simulink model "PMSM_RobotKinematics"  (R2018b)
settings: Solver=VariableStepAuto  StartTime=0.0  StopTime=0.2  FixedStep=Ts  RelTol=1e-4  EnableMultiTasking=on
PreLoadFcn:
  | run('Arm6Assembly_DataFile.m');
model workspace: external: MAT-File E:\SixRobotArm\Simscape_Simulation\StepFile\Arm6Assembly_DataFile.mat (data not in the file)
values from neighbouring files (symbols this model uses):
  smiData =     [Arm6SimscapeData.mat]
undefined symbols (not defined in the file or in its folder): X, Y, Z
libraries: sm_lib x36, fl_lib x25, nesl_utility x19, simulink_extras x7
(part 2 of 4)

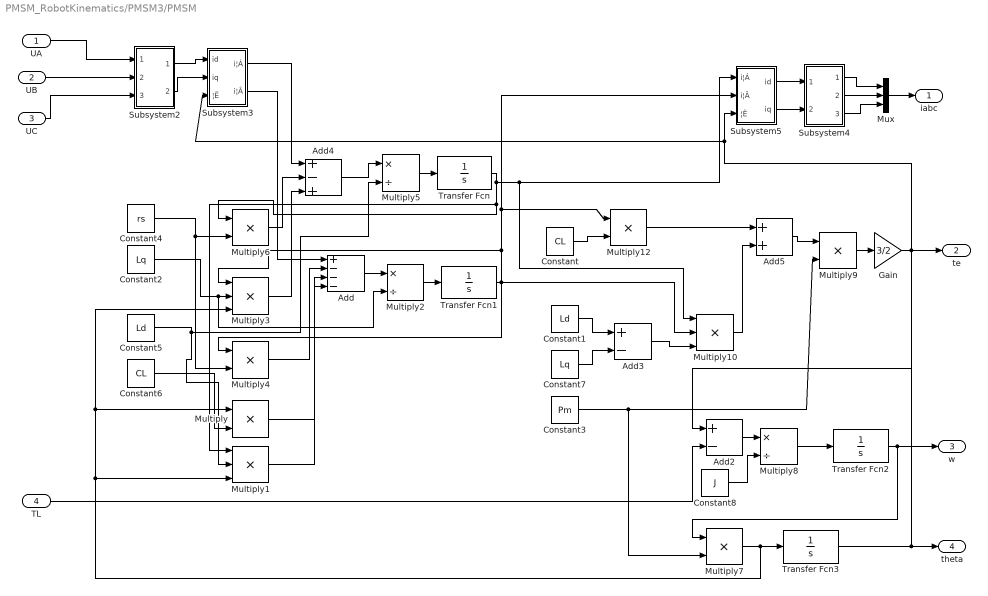
== system PMSM_RobotKinematics/PMSM3/PMSM ==
  UA : Inport
  UB : Inport  Port=2
  UC : Inport  Port=3
  TL : Inport  Port=4
  Add : Sum  Inputs=+---  SaturateOnIntegerOverflow=on  OutDataTypeStr=Inherit: Same as first input
  Add2 : Sum  Inputs=+-  SaturateOnIntegerOverflow=on  InputSameDT=on  OutDataTypeStr=Inherit: Same as first input
  Add3 : Sum  Inputs=+-  SaturateOnIntegerOverflow=on  InputSameDT=on  OutDataTypeStr=Inherit: Same as first input
  Add4 : Sum  Inputs=+-+  SaturateOnIntegerOverflow=on  InputSameDT=on  OutDataTypeStr=Inherit: Same as first input
  Add5 : Sum  SaturateOnIntegerOverflow=on  InputSameDT=on  OutDataTypeStr=Inherit: Same as first input
  Constant : Constant  Value=CL
  Constant1 : Constant  Value=Ld
  Constant2 : Constant  Value=Lq
  Constant3 : Constant  Value=Pm
  Constant4 : Constant  Value=rs
  Constant5 : Constant  Value=Ld
  Constant6 : Constant  Value=CL
  Constant7 : Constant  Value=Lq
  Constant8 : Constant  Value=J
  Gain : Gain  Gain=3/2  SaturateOnIntegerOverflow=on  OutDataTypeStr=Inherit: Same as input  ParamDataTypeStr=Inherit: Same as input
  Multiply{,4,6..7,9,12} (6 alike) : Product  Inputs=**  SaturateOnIntegerOverflow=on  OutDataTypeStr=Inherit: Same as first input
  Multiply1 : Product  Inputs=***  SaturateOnIntegerOverflow=on  OutDataTypeStr=Inherit: Same as first input
  Multiply10 : Product  Inputs=***  SaturateOnIntegerOverflow=on  OutDataTypeStr=Inherit: Same as first input
  Multiply2 : Product  Inputs=*/  SaturateOnIntegerOverflow=on  OutDataTypeStr=Inherit: Same as first input
  Multiply3 : Product  Inputs=***  SaturateOnIntegerOverflow=on  OutDataTypeStr=Inherit: Same as first input
  Multiply5 : Product  Inputs=*/  SaturateOnIntegerOverflow=on  OutDataTypeStr=Inherit: Same as first input
  Multiply8 : Product  Inputs=*/  SaturateOnIntegerOverflow=on  OutDataTypeStr=Inherit: Same as first input
  Mux : Mux  Inputs=3
  Subsystem2 : Subsystem  mask(hao){}
      mask help: 3/2
      mask Help: no
      mask Display: disp('3/2')
  Subsystem3 : Subsystem  mask(2/2){}
      mask help: qdtoMT
      mask Help: none
  Subsystem4 : Subsystem  mask(hao){}
      mask help: 2/3
      mask Help: npi
      mask Display: disp('2/3')
  Subsystem5 : Subsystem  mask(2/2){}
      mask help: mt-todq
      mask Help: no
  Transfer Fcn : TransferFcn  Denominator=[1 0]  AbsoluteTolerance=1e-3
  Transfer Fcn1 : TransferFcn  Denominator=[1 0]
  Transfer Fcn2 : TransferFcn  Denominator=[1 0]
  Transfer Fcn3 : TransferFcn  Denominator=[1 0]
  iabc : Outport
  te : Outport  Port=2
  w : Outport  Port=3
  theta : Outport  Port=4
  wires:
  Multiply2/1 -> Transfer Fcn1/1
  Multiply5/1 -> Transfer Fcn/1
  TL/1 -> Add2/2
  Constant8/1 -> Multiply8/2
  Add2/1 -> Multiply8/1
  Subsystem5/2(iq) -> Subsystem4/2(In3)
  Subsystem5/1(id) -> Subsystem4/1(In1)
  Constant3/1 -> Multiply7/2, Multiply9/2
  Multiply10/1 -> Add5/2
  Multiply12/1 -> Add5/1
  Constant7/1 -> Add3/2
  Constant1/1 -> Add3/1
  Multiply1/1 -> Add/4
  Multiply/1 -> Add/3
  Multiply4/1 -> Add/2
  Add/1 -> Multiply2/1
  Subsystem3/2(i¦Â) -> Add/1
  Add4/1 -> Multiply5/1
  Multiply3/1 -> Add4/3
  Multiply6/1 -> Add4/2
  Subsystem3/1(i¦Á) -> Add4/1
  Subsystem2/2(Out2) -> Subsystem3/2(iq)
  Subsystem2/1(Out1) -> Subsystem3/1(id)
  Transfer Fcn/1 -> Multiply6/1, Multiply1/1, Multiply10/1, Subsystem5/1(i¦Á)
  Constant4/1 -> Multiply6/2, Multiply4/2
  Transfer Fcn1/1 -> Multiply3/1, Multiply12/1, Subsystem5/2(i¦Â), Multiply4/1, Multiply10/2
  Constant2/1 -> Multiply3/2, Multiply2/2
  Constant5/1 -> Multiply1/2, Multiply5/2
  Constant6/1 -> Multiply/2
  Multiply7/1 -> Transfer Fcn3/1, Multiply3/3, Multiply/1, Multiply1/3
  Constant/1 -> Multiply12/2
  Add3/1 -> Multiply10/3
  Transfer Fcn2/1 -> Multiply7/1, w/1
  Add5/1 -> Multiply9/1
  Multiply9/1 -> Gain/1
  Subsystem4/3(Out3) -> Mux/3
  Mux/1 -> iabc/1
  Multiply8/1 -> Transfer Fcn2/1
  UC/1 -> Subsystem2/3(In3)
  Transfer Fcn3/1 -> Subsystem5/3(¦Ë), Subsystem3/3(¦Ë), theta/1
  Gain/1 -> te/1, Add2/1
  Subsystem4/1(Out1) -> Mux/1
  Subsystem4/2(Out2) -> Mux/2
  UA/1 -> Subsystem2/1(In1)
  UB/1 -> Subsystem2/2(In2)

== system PMSM_RobotKinematics/PMSM3/Park ==
  I_alpha : Inport
  I_beta : Inport  Port=2
  Theta : Inport  Port=3
  Fcn : Fcn  Expr=sin(u)
  Fcn1 : Fcn  Expr=cos(u)
  Gain : Gain  SaturateOnIntegerOverflow=on  OutDataTypeStr=Inherit: Same as input  ParamDataTypeStr=Inherit: Same as input
  Gain1 : Gain  SaturateOnIntegerOverflow=on  OutDataTypeStr=Inherit: Same as input  ParamDataTypeStr=Inherit: Same as input
  Mux : Mux  Inputs=[1 1 1 1]
  id : Fcn  Expr=u[1]*u[3]+u[2]*u[4]
  iq : Fcn  Expr=-u[2]*u[3]+u[1]*u[4]
  Id : Outport  InitialOutput=0
  Iq : Outport  Port=2  InitialOutput=0
  wires:
  Fcn/1 -> Mux/2
  Fcn1/1 -> Mux/1
  Theta/1 -> Fcn1/1, Fcn/1
  Mux/1 -> iq/1, id/1
  I_alpha/1 -> Mux/3
  iq/1 -> Gain1/1
  id/1 -> Gain/1
  Gain/1 -> Id/1
  Gain1/1 -> Iq/1
  I_beta/1 -> Mux/4

== system PMSM_RobotKinematics/PMSM3/Park_inv ==
  iq : Inport
  id : Inport  Port=2
  Theta : Inport  Port=3
  Fcn : Fcn  Expr=sin(u)
  Fcn1 : Fcn  Expr=cos(u)
  Gain : Gain  SaturateOnIntegerOverflow=on  OutDataTypeStr=Inherit: Same as input  ParamDataTypeStr=Inherit: Same as input
  Gain1 : Gain  SaturateOnIntegerOverflow=on  OutDataTypeStr=Inherit: Same as input  ParamDataTypeStr=Inherit: Same as input
  Mux : Mux  Inputs=[1 1 1 1]
  i_alpha : Fcn  Expr=u[1]*u[4]-u[2]*u[3]
  i_beta : Fcn  Expr=u[2]*u[4]+u[1]*u[3]
  I_apha : Outport  InitialOutput=0
  I_beta : Outport  Port=2  InitialOutput=0
  wires:
  Fcn/1 -> Mux/2
  Fcn1/1 -> Mux/1
  Theta/1 -> Fcn1/1, Fcn/1
  Mux/1 -> i_beta/1, i_alpha/1
  iq/1 -> Mux/3
  i_beta/1 -> Gain1/1
  i_alpha/1 -> Gain/1
  Gain/1 -> I_apha/1
  Gain1/1 -> I_beta/1
  id/1 -> Mux/4

== system PMSM_RobotKinematics/PMSM3/iqref ==
  In_1 : Inport
  Integral : TransferFcn  Numerator=[I]  Denominator=[1 0]
  Proportional : Gain  Gain=P  SaturateOnIntegerOverflow=on  OutDataTypeStr=Inherit: Same as input  ParamDataTypeStr=Inherit: Same as input
  Saturation : Saturate  UpperLimit=max  LowerLimit=min
  Sum : Sum  SaturateOnIntegerOverflow=on  InputSameDT=on  OutDataTypeStr=Inherit: Same as first input
  Out_1 : Outport  InitialOutput=0
  wires:
  Integral/1 -> Sum/2
  In_1/1 -> Integral/1, Proportional/1
  Proportional/1 -> Sum/1
  Sum/1 -> Saturation/1
  Saturation/1 -> Out_1/1

== system PMSM_RobotKinematics/PMSM3/iqref1 ==
  In_1 : Inport
  Integral : TransferFcn  Numerator=[I]  Denominator=[1 0]
  Proportional : Gain  Gain=P  SaturateOnIntegerOverflow=on  OutDataTypeStr=Inherit: Same as input  ParamDataTypeStr=Inherit: Same as input
  Saturation : Saturate  UpperLimit=max  LowerLimit=min
  Sum : Sum  SaturateOnIntegerOverflow=on  InputSameDT=on  OutDataTypeStr=Inherit: Same as first input
  Out_1 : Outport  InitialOutput=0
  wires:
  Saturation/1 -> Out_1/1
  Sum/1 -> Saturation/1
  Proportional/1 -> Sum/1
  In_1/1 -> Proportional/1, Integral/1
  Integral/1 -> Sum/2

== system PMSM_RobotKinematics/PMSM3/iqref2 ==
  In_1 : Inport
  Integral : TransferFcn  Numerator=[I]  Denominator=[1 0]
  Proportional : Gain  Gain=P  SaturateOnIntegerOverflow=on  OutDataTypeStr=Inherit: Same as input  ParamDataTypeStr=Inherit: Same as input
  Saturation : Saturate  UpperLimit=max  LowerLimit=min
  Sum : Sum  SaturateOnIntegerOverflow=on  InputSameDT=on  OutDataTypeStr=Inherit: Same as first input
  Out_1 : Outport  InitialOutput=0
  wires:
  Saturation/1 -> Out_1/1
  Sum/1 -> Saturation/1
  Proportional/1 -> Sum/1
  In_1/1 -> Proportional/1, Integral/1
  Integral/1 -> Sum/2

== system PMSM_RobotKinematics/PMSM3/iqref3 ==
  In_1 : Inport
  Integral : TransferFcn  Numerator=[I]  Denominator=[1 0]
  Proportional : Gain  Gain=P  SaturateOnIntegerOverflow=on  OutDataTypeStr=Inherit: Same as input  ParamDataTypeStr=Inherit: Same as input
  Saturation : Saturate  UpperLimit=max  LowerLimit=min
  Sum : Sum  SaturateOnIntegerOverflow=on  InputSameDT=on  OutDataTypeStr=Inherit: Same as first input
  Out_1 : Outport  InitialOutput=0
  wires:
  Integral/1 -> Sum/2
  In_1/1 -> Integral/1, Proportional/1
  Proportional/1 -> Sum/1
  Sum/1 -> Saturation/1
  Saturation/1 -> Out_1/1

== system PMSM_RobotKinematics/PMSM4/Clarke ==
  is_abc : Inport
  Gain : Gain  Gain=sqrt(3/2)  SaturateOnIntegerOverflow=on  OutDataTypeStr=Inherit: Same as input  ParamDataTypeStr=Inherit: Same as input
  Gain1 : Gain  Gain=sqrt(2)/2  SaturateOnIntegerOverflow=on  OutDataTypeStr=Inherit: Same as input  ParamDataTypeStr=Inherit: Same as input
  Mux : Mux  Inputs=[3]
  i_alpha : Fcn  Expr=u[1]
  i_beta : Fcn  Expr=u[1]+2*u[2]
  I_alpha : Outport  InitialOutput=0
  I_beta : Outport  Port=2  InitialOutput=0
  wires:
  Gain1/1 -> I_beta/1
  Gain/1 -> I_alpha/1
  i_alpha/1 -> Gain/1
  i_beta/1 -> Gain1/1
  is_abc/1 -> Mux/1
  Mux/1 -> i_alpha/1, i_beta/1

== system PMSM_RobotKinematics/PMSM4/Clarke_inv ==
  Valpha : Inport
  Vbeta : Inport  Port=2
  Fcn : Fcn  Expr=-u[1]/2+1.73205081*u[2]/2
  Fcn1 : Fcn  Expr=-u[1]/2-1.73205081*u[2]/2
  Gain1 : Gain  Gain=sqrt(2/3)  SaturateOnIntegerOverflow=on  OutDataTypeStr=Inherit: Same as input  ParamDataTypeStr=Inherit: Same as input
  Gain2 : Gain  Gain=sqrt(2/3)  SaturateOnIntegerOverflow=on  OutDataTypeStr=Inherit: Same as input  ParamDataTypeStr=Inherit: Same as input
  Gain3 : Gain  Gain=sqrt(2/3)  SaturateOnIntegerOverflow=on  OutDataTypeStr=Inherit: Same as input  ParamDataTypeStr=Inherit: Same as input
  Mux : Mux  Inputs=2
  Va : Outport
  Vb : Outport  Port=2
  Vc : Outport  Port=3
  wires:
  Gain3/1 -> Vc/1
  Gain2/1 -> Vb/1
  Gain1/1 -> Va/1
  Vbeta/1 -> Mux/2
  Valpha/1 -> Gain1/1, Mux/1
  Fcn1/1 -> Gain3/1
  Fcn/1 -> Gain2/1
  Mux/1 -> Fcn1/1, Fcn/1

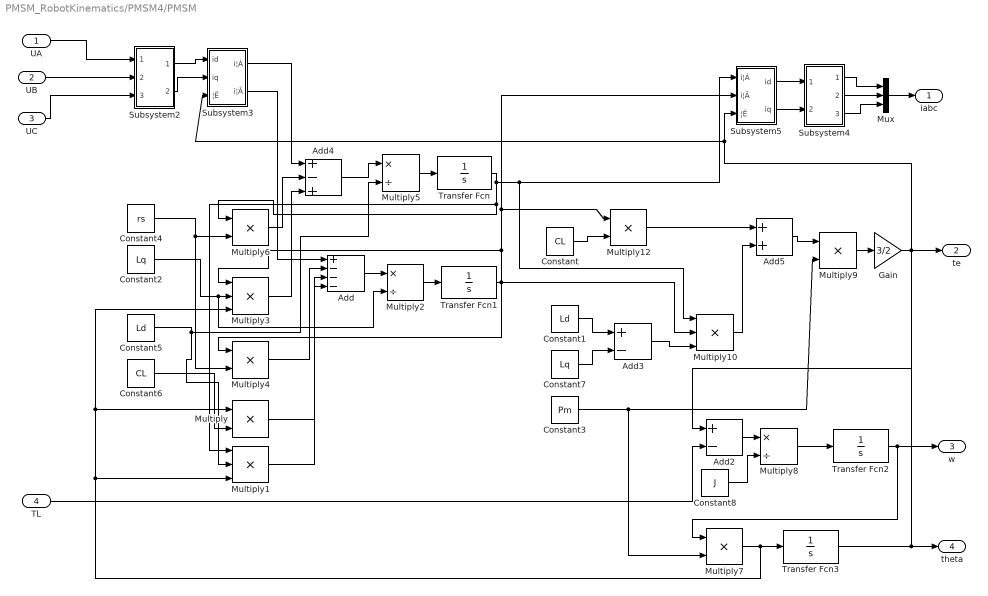
== system PMSM_RobotKinematics/PMSM4/PMSM ==
  UA : Inport
  UB : Inport  Port=2
  UC : Inport  Port=3
  TL : Inport  Port=4
  Add : Sum  Inputs=+---  SaturateOnIntegerOverflow=on  OutDataTypeStr=Inherit: Same as first input
  Add2 : Sum  Inputs=+-  SaturateOnIntegerOverflow=on  InputSameDT=on  OutDataTypeStr=Inherit: Same as first input
  Add3 : Sum  Inputs=+-  SaturateOnIntegerOverflow=on  InputSameDT=on  OutDataTypeStr=Inherit: Same as first input
  Add4 : Sum  Inputs=+-+  SaturateOnIntegerOverflow=on  InputSameDT=on  OutDataTypeStr=Inherit: Same as first input
  Add5 : Sum  SaturateOnIntegerOverflow=on  InputSameDT=on  OutDataTypeStr=Inherit: Same as first input
  Constant : Constant  Value=CL
  Constant1 : Constant  Value=Ld
  Constant2 : Constant  Value=Lq
  Constant3 : Constant  Value=Pm
  Constant4 : Constant  Value=rs
  Constant5 : Constant  Value=Ld
  Constant6 : Constant  Value=CL
  Constant7 : Constant  Value=Lq
  Constant8 : Constant  Value=J
  Gain : Gain  Gain=3/2  SaturateOnIntegerOverflow=on  OutDataTypeStr=Inherit: Same as input  ParamDataTypeStr=Inherit: Same as input
  Multiply{,4,6..7,9,12} (6 alike) : Product  Inputs=**  SaturateOnIntegerOverflow=on  OutDataTypeStr=Inherit: Same as first input
  Multiply1 : Product  Inputs=***  SaturateOnIntegerOverflow=on  OutDataTypeStr=Inherit: Same as first input
  Multiply10 : Product  Inputs=***  SaturateOnIntegerOverflow=on  OutDataTypeStr=Inherit: Same as first input
  Multiply2 : Product  Inputs=*/  SaturateOnIntegerOverflow=on  OutDataTypeStr=Inherit: Same as first input
  Multiply3 : Product  Inputs=***  SaturateOnIntegerOverflow=on  OutDataTypeStr=Inherit: Same as first input
  Multiply5 : Product  Inputs=*/  SaturateOnIntegerOverflow=on  OutDataTypeStr=Inherit: Same as first input
  Multiply8 : Product  Inputs=*/  SaturateOnIntegerOverflow=on  OutDataTypeStr=Inherit: Same as first input
  Mux : Mux  Inputs=3
  Subsystem2 : Subsystem  mask(hao){}
      mask help: 3/2
      mask Help: no
      mask Display: disp('3/2')
  Subsystem3 : Subsystem  mask(2/2){}
      mask help: qdtoMT
      mask Help: none
  Subsystem4 : Subsystem  mask(hao){}
      mask help: 2/3
      mask Help: npi
      mask Display: disp('2/3')
  Subsystem5 : Subsystem  mask(2/2){}
      mask help: mt-todq
      mask Help: no
  Transfer Fcn : TransferFcn  Denominator=[1 0]  AbsoluteTolerance=1e-3
  Transfer Fcn1 : TransferFcn  Denominator=[1 0]
  Transfer Fcn2 : TransferFcn  Denominator=[1 0]
  Transfer Fcn3 : TransferFcn  Denominator=[1 0]
  iabc : Outport
  te : Outport  Port=2
  w : Outport  Port=3
  theta : Outport  Port=4
  wires:
  UB/1 -> Subsystem2/2(In2)
  UA/1 -> Subsystem2/1(In1)
  Subsystem4/2(Out2) -> Mux/2
  Subsystem4/1(Out1) -> Mux/1
  Gain/1 -> Add2/1, te/1
  Transfer Fcn3/1 -> theta/1, Subsystem3/3(¦Ë), Subsystem5/3(¦Ë)
  UC/1 -> Subsystem2/3(In3)
  Multiply8/1 -> Transfer Fcn2/1
  Mux/1 -> iabc/1
  Subsystem4/3(Out3) -> Mux/3
  Multiply9/1 -> Gain/1
  Add5/1 -> Multiply9/1
  Transfer Fcn2/1 -> w/1, Multiply7/1
  Add3/1 -> Multiply10/3
  Constant/1 -> Multiply12/2
  Multiply7/1 -> Multiply1/3, Multiply/1, Multiply3/3, Transfer Fcn3/1
  Constant6/1 -> Multiply/2
  Constant5/1 -> Multiply5/2, Multiply1/2
  Constant2/1 -> Multiply2/2, Multiply3/2
  Transfer Fcn1/1 -> Multiply10/2, Multiply4/1, Subsystem5/2(i¦Â), Multiply12/1, Multiply3/1
  Constant4/1 -> Multiply4/2, Multiply6/2
  Transfer Fcn/1 -> Subsystem5/1(i¦Á), Multiply10/1, Multiply1/1, Multiply6/1
  Subsystem2/1(Out1) -> Subsystem3/1(id)
  Subsystem2/2(Out2) -> Subsystem3/2(iq)
  Subsystem3/1(i¦Á) -> Add4/1
  Multiply6/1 -> Add4/2
  Multiply3/1 -> Add4/3
  Add4/1 -> Multiply5/1
  Subsystem3/2(i¦Â) -> Add/1
  Add/1 -> Multiply2/1
  Multiply4/1 -> Add/2
  Multiply/1 -> Add/3
  Multiply1/1 -> Add/4
  Constant1/1 -> Add3/1
  Constant7/1 -> Add3/2
  Multiply12/1 -> Add5/1
  Multiply10/1 -> Add5/2
  Constant3/1 -> Multiply9/2, Multiply7/2
  Subsystem5/1(id) -> Subsystem4/1(In1)
  Subsystem5/2(iq) -> Subsystem4/2(In3)
  Add2/1 -> Multiply8/1
  Constant8/1 -> Multiply8/2
  TL/1 -> Add2/2
  Multiply5/1 -> Transfer Fcn/1
  Multiply2/1 -> Transfer Fcn1/1

== system PMSM_RobotKinematics/PMSM4/Park ==
  I_alpha : Inport
  I_beta : Inport  Port=2
  Theta : Inport  Port=3
  Fcn : Fcn  Expr=sin(u)
  Fcn1 : Fcn  Expr=cos(u)
  Gain : Gain  SaturateOnIntegerOverflow=on  OutDataTypeStr=Inherit: Same as input  ParamDataTypeStr=Inherit: Same as input
  Gain1 : Gain  SaturateOnIntegerOverflow=on  OutDataTypeStr=Inherit: Same as input  ParamDataTypeStr=Inherit: Same as input
  Mux : Mux  Inputs=[1 1 1 1]
  id : Fcn  Expr=u[1]*u[3]+u[2]*u[4]
  iq : Fcn  Expr=-u[2]*u[3]+u[1]*u[4]
  Id : Outport  InitialOutput=0
  Iq : Outport  Port=2  InitialOutput=0
  wires:
  I_beta/1 -> Mux/4
  Gain1/1 -> Iq/1
  Gain/1 -> Id/1
  id/1 -> Gain/1
  iq/1 -> Gain1/1
  I_alpha/1 -> Mux/3
  Mux/1 -> id/1, iq/1
  Theta/1 -> Fcn/1, Fcn1/1
  Fcn1/1 -> Mux/1
  Fcn/1 -> Mux/2

== system PMSM_RobotKinematics/PMSM4/Park_inv ==
  iq : Inport
  id : Inport  Port=2
  Theta : Inport  Port=3
  Fcn : Fcn  Expr=sin(u)
  Fcn1 : Fcn  Expr=cos(u)
  Gain : Gain  SaturateOnIntegerOverflow=on  OutDataTypeStr=Inherit: Same as input  ParamDataTypeStr=Inherit: Same as input
  Gain1 : Gain  SaturateOnIntegerOverflow=on  OutDataTypeStr=Inherit: Same as input  ParamDataTypeStr=Inherit: Same as input
  Mux : Mux  Inputs=[1 1 1 1]
  i_alpha : Fcn  Expr=u[1]*u[4]-u[2]*u[3]
  i_beta : Fcn  Expr=u[2]*u[4]+u[1]*u[3]
  I_apha : Outport  InitialOutput=0
  I_beta : Outport  Port=2  InitialOutput=0
  wires:
  id/1 -> Mux/4
  Gain1/1 -> I_beta/1
  Gain/1 -> I_apha/1
  i_alpha/1 -> Gain/1
  i_beta/1 -> Gain1/1
  iq/1 -> Mux/3
  Mux/1 -> i_alpha/1, i_beta/1
  Theta/1 -> Fcn/1, Fcn1/1
  Fcn1/1 -> Mux/1
  Fcn/1 -> Mux/2

== system PMSM_RobotKinematics/PMSM4/iqref ==
  In_1 : Inport
  Integral : TransferFcn  Numerator=[I]  Denominator=[1 0]
  Proportional : Gain  Gain=P  SaturateOnIntegerOverflow=on  OutDataTypeStr=Inherit: Same as input  ParamDataTypeStr=Inherit: Same as input
  Saturation : Saturate  UpperLimit=max  LowerLimit=min
  Sum : Sum  SaturateOnIntegerOverflow=on  InputSameDT=on  OutDataTypeStr=Inherit: Same as first input
  Out_1 : Outport  InitialOutput=0
  wires:
  Saturation/1 -> Out_1/1
  Sum/1 -> Saturation/1
  Proportional/1 -> Sum/1
  In_1/1 -> Proportional/1, Integral/1
  Integral/1 -> Sum/2

== system PMSM_RobotKinematics/PMSM4/iqref1 ==
  In_1 : Inport
  Integral : TransferFcn  Numerator=[I]  Denominator=[1 0]
  Proportional : Gain  Gain=P  SaturateOnIntegerOverflow=on  OutDataTypeStr=Inherit: Same as input  ParamDataTypeStr=Inherit: Same as input
  Saturation : Saturate  UpperLimit=max  LowerLimit=min
  Sum : Sum  SaturateOnIntegerOverflow=on  InputSameDT=on  OutDataTypeStr=Inherit: Same as first input
  Out_1 : Outport  InitialOutput=0
  wires:
  Integral/1 -> Sum/2
  In_1/1 -> Integral/1, Proportional/1
  Proportional/1 -> Sum/1
  Sum/1 -> Saturation/1
  Saturation/1 -> Out_1/1

== system PMSM_RobotKinematics/PMSM4/iqref2 ==
  In_1 : Inport
  Integral : TransferFcn  Numerator=[I]  Denominator=[1 0]
  Proportional : Gain  Gain=P  SaturateOnIntegerOverflow=on  OutDataTypeStr=Inherit: Same as input  ParamDataTypeStr=Inherit: Same as input
  Saturation : Saturate  UpperLimit=max  LowerLimit=min
  Sum : Sum  SaturateOnIntegerOverflow=on  InputSameDT=on  OutDataTypeStr=Inherit: Same as first input
  Out_1 : Outport  InitialOutput=0
  wires:
  Integral/1 -> Sum/2
  In_1/1 -> Integral/1, Proportional/1
  Proportional/1 -> Sum/1
  Sum/1 -> Saturation/1
  Saturation/1 -> Out_1/1

== system PMSM_RobotKinematics/PMSM4/iqref3 ==
  In_1 : Inport
  Integral : TransferFcn  Numerator=[I]  Denominator=[1 0]
  Proportional : Gain  Gain=P  SaturateOnIntegerOverflow=on  OutDataTypeStr=Inherit: Same as input  ParamDataTypeStr=Inherit: Same as input
  Saturation : Saturate  UpperLimit=max  LowerLimit=min
  Sum : Sum  SaturateOnIntegerOverflow=on  InputSameDT=on  OutDataTypeStr=Inherit: Same as first input
  Out_1 : Outport  InitialOutput=0
  wires:
  Saturation/1 -> Out_1/1
  Sum/1 -> Saturation/1
  Proportional/1 -> Sum/1
  In_1/1 -> Proportional/1, Integral/1
  Integral/1 -> Sum/2

== system PMSM_RobotKinematics/PMSM5/Clarke ==
  is_abc : Inport
  Gain : Gain  Gain=sqrt(3/2)  SaturateOnIntegerOverflow=on  OutDataTypeStr=Inherit: Same as input  ParamDataTypeStr=Inherit: Same as input
  Gain1 : Gain  Gain=sqrt(2)/2  SaturateOnIntegerOverflow=on  OutDataTypeStr=Inherit: Same as input  ParamDataTypeStr=Inherit: Same as input
  Mux : Mux  Inputs=[3]
  i_alpha : Fcn  Expr=u[1]
  i_beta : Fcn  Expr=u[1]+2*u[2]
  I_alpha : Outport  InitialOutput=0
  I_beta : Outport  Port=2  InitialOutput=0
  wires:
  Mux/1 -> i_beta/1, i_alpha/1
  is_abc/1 -> Mux/1
  i_beta/1 -> Gain1/1
  i_alpha/1 -> Gain/1
  Gain/1 -> I_alpha/1
  Gain1/1 -> I_beta/1

== system PMSM_RobotKinematics/PMSM5/Clarke_inv ==
  Valpha : Inport
  Vbeta : Inport  Port=2
  Fcn : Fcn  Expr=-u[1]/2+1.73205081*u[2]/2
  Fcn1 : Fcn  Expr=-u[1]/2-1.73205081*u[2]/2
  Gain1 : Gain  Gain=sqrt(2/3)  SaturateOnIntegerOverflow=on  OutDataTypeStr=Inherit: Same as input  ParamDataTypeStr=Inherit: Same as input
  Gain2 : Gain  Gain=sqrt(2/3)  SaturateOnIntegerOverflow=on  OutDataTypeStr=Inherit: Same as input  ParamDataTypeStr=Inherit: Same as input
  Gain3 : Gain  Gain=sqrt(2/3)  SaturateOnIntegerOverflow=on  OutDataTypeStr=Inherit: Same as input  ParamDataTypeStr=Inherit: Same as input
  Mux : Mux  Inputs=2
  Va : Outport
  Vb : Outport  Port=2
  Vc : Outport  Port=3
  wires:
  Mux/1 -> Fcn/1, Fcn1/1
  Fcn/1 -> Gain2/1
  Fcn1/1 -> Gain3/1
  Valpha/1 -> Mux/1, Gain1/1
  Vbeta/1 -> Mux/2
  Gain1/1 -> Va/1
  Gain2/1 -> Vb/1
  Gain3/1 -> Vc/1

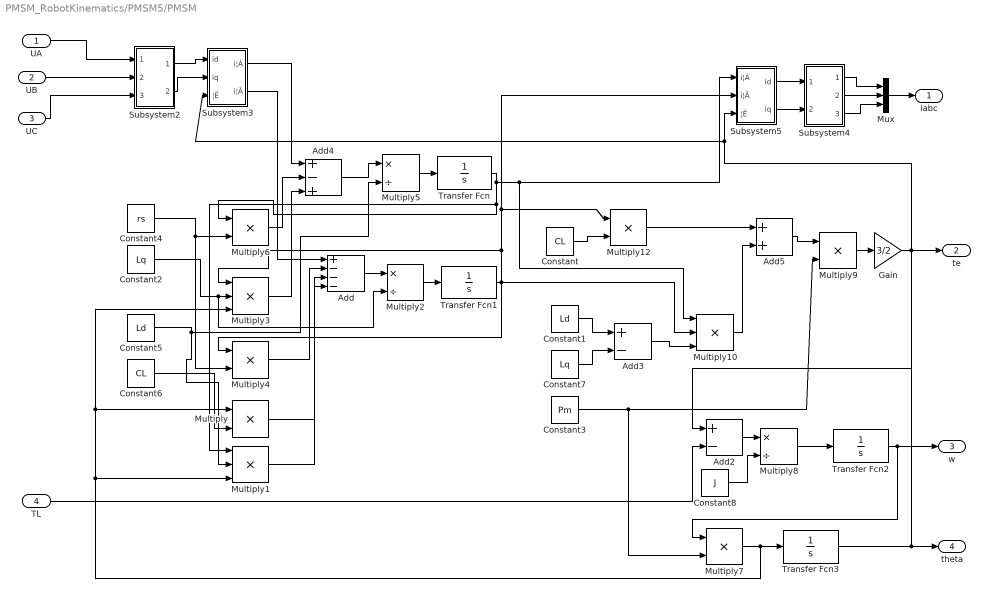
== system PMSM_RobotKinematics/PMSM5/PMSM ==
  UA : Inport
  UB : Inport  Port=2
  UC : Inport  Port=3
  TL : Inport  Port=4
  Add : Sum  Inputs=+---  SaturateOnIntegerOverflow=on  OutDataTypeStr=Inherit: Same as first input
  Add2 : Sum  Inputs=+-  SaturateOnIntegerOverflow=on  InputSameDT=on  OutDataTypeStr=Inherit: Same as first input
  Add3 : Sum  Inputs=+-  SaturateOnIntegerOverflow=on  InputSameDT=on  OutDataTypeStr=Inherit: Same as first input
  Add4 : Sum  Inputs=+-+  SaturateOnIntegerOverflow=on  InputSameDT=on  OutDataTypeStr=Inherit: Same as first input
  Add5 : Sum  SaturateOnIntegerOverflow=on  InputSameDT=on  OutDataTypeStr=Inherit: Same as first input
  Constant : Constant  Value=CL
  Constant1 : Constant  Value=Ld
  Constant2 : Constant  Value=Lq
  Constant3 : Constant  Value=Pm
  Constant4 : Constant  Value=rs
  Constant5 : Constant  Value=Ld
  Constant6 : Constant  Value=CL
  Constant7 : Constant  Value=Lq
  Constant8 : Constant  Value=J
  Gain : Gain  Gain=3/2  SaturateOnIntegerOverflow=on  OutDataTypeStr=Inherit: Same as input  ParamDataTypeStr=Inherit: Same as input
  Multiply{,4,6..7,9,12} (6 alike) : Product  Inputs=**  SaturateOnIntegerOverflow=on  OutDataTypeStr=Inherit: Same as first input
  Multiply1 : Product  Inputs=***  SaturateOnIntegerOverflow=on  OutDataTypeStr=Inherit: Same as first input
  Multiply10 : Product  Inputs=***  SaturateOnIntegerOverflow=on  OutDataTypeStr=Inherit: Same as first input
  Multiply2 : Product  Inputs=*/  SaturateOnIntegerOverflow=on  OutDataTypeStr=Inherit: Same as first input
  Multiply3 : Product  Inputs=***  SaturateOnIntegerOverflow=on  OutDataTypeStr=Inherit: Same as first input
  Multiply5 : Product  Inputs=*/  SaturateOnIntegerOverflow=on  OutDataTypeStr=Inherit: Same as first input
  Multiply8 : Product  Inputs=*/  SaturateOnIntegerOverflow=on  OutDataTypeStr=Inherit: Same as first input
  Mux : Mux  Inputs=3
  Subsystem2 : Subsystem  mask(hao){}
      mask help: 3/2
      mask Help: no
      mask Display: disp('3/2')
  Subsystem3 : Subsystem  mask(2/2){}
      mask help: qdtoMT
      mask Help: none
  Subsystem4 : Subsystem  mask(hao){}
      mask help: 2/3
      mask Help: npi
      mask Display: disp('2/3')
  Subsystem5 : Subsystem  mask(2/2){}
      mask help: mt-todq
      mask Help: no
  Transfer Fcn : TransferFcn  Denominator=[1 0]  AbsoluteTolerance=1e-3
  Transfer Fcn1 : TransferFcn  Denominator=[1 0]
  Transfer Fcn2 : TransferFcn  Denominator=[1 0]
  Transfer Fcn3 : TransferFcn  Denominator=[1 0]
  iabc : Outport
  te : Outport  Port=2
  w : Outport  Port=3
  theta : Outport  Port=4
  wires:
  Multiply2/1 -> Transfer Fcn1/1
  Multiply5/1 -> Transfer Fcn/1
  TL/1 -> Add2/2
  Constant8/1 -> Multiply8/2
  Add2/1 -> Multiply8/1
  Subsystem5/2(iq) -> Subsystem4/2(In3)
  Subsystem5/1(id) -> Subsystem4/1(In1)
  Constant3/1 -> Multiply7/2, Multiply9/2
  Multiply10/1 -> Add5/2
  Multiply12/1 -> Add5/1
  Constant7/1 -> Add3/2
  Constant1/1 -> Add3/1
  Multiply1/1 -> Add/4
  Multiply/1 -> Add/3
  Multiply4/1 -> Add/2
  Add/1 -> Multiply2/1
  Subsystem3/2(i¦Â) -> Add/1
  Add4/1 -> Multiply5/1
  Multiply3/1 -> Add4/3
  Multiply6/1 -> Add4/2
  Subsystem3/1(i¦Á) -> Add4/1
  Subsystem2/2(Out2) -> Subsystem3/2(iq)
  Subsystem2/1(Out1) -> Subsystem3/1(id)
  Transfer Fcn/1 -> Multiply6/1, Multiply1/1, Multiply10/1, Subsystem5/1(i¦Á)
  Constant4/1 -> Multiply6/2, Multiply4/2
  Transfer Fcn1/1 -> Multiply3/1, Multiply12/1, Subsystem5/2(i¦Â), Multiply4/1, Multiply10/2
  Constant2/1 -> Multiply3/2, Multiply2/2
  Constant5/1 -> Multiply1/2, Multiply5/2
  Constant6/1 -> Multiply/2
  Multiply7/1 -> Transfer Fcn3/1, Multiply3/3, Multiply/1, Multiply1/3
  Constant/1 -> Multiply12/2
  Add3/1 -> Multiply10/3
  Transfer Fcn2/1 -> Multiply7/1, w/1
  Add5/1 -> Multiply9/1
  Multiply9/1 -> Gain/1
  Subsystem4/3(Out3) -> Mux/3
  Mux/1 -> iabc/1
  Multiply8/1 -> Transfer Fcn2/1
  UC/1 -> Subsystem2/3(In3)
  Transfer Fcn3/1 -> Subsystem5/3(¦Ë), Subsystem3/3(¦Ë), theta/1
  Gain/1 -> te/1, Add2/1
  Subsystem4/1(Out1) -> Mux/1
  Subsystem4/2(Out2) -> Mux/2
  UA/1 -> Subsystem2/1(In1)
  UB/1 -> Subsystem2/2(In2)

== system PMSM_RobotKinematics/PMSM5/Park ==
  I_alpha : Inport
  I_beta : Inport  Port=2
  Theta : Inport  Port=3
  Fcn : Fcn  Expr=sin(u)
  Fcn1 : Fcn  Expr=cos(u)
  Gain : Gain  SaturateOnIntegerOverflow=on  OutDataTypeStr=Inherit: Same as input  ParamDataTypeStr=Inherit: Same as input
  Gain1 : Gain  SaturateOnIntegerOverflow=on  OutDataTypeStr=Inherit: Same as input  ParamDataTypeStr=Inherit: Same as input
  Mux : Mux  Inputs=[1 1 1 1]
  id : Fcn  Expr=u[1]*u[3]+u[2]*u[4]
  iq : Fcn  Expr=-u[2]*u[3]+u[1]*u[4]
  Id : Outport  InitialOutput=0
  Iq : Outport  Port=2  InitialOutput=0
  wires:
  Fcn/1 -> Mux/2
  Fcn1/1 -> Mux/1
  Theta/1 -> Fcn1/1, Fcn/1
  Mux/1 -> iq/1, id/1
  I_alpha/1 -> Mux/3
  iq/1 -> Gain1/1
  id/1 -> Gain/1
  Gain/1 -> Id/1
  Gain1/1 -> Iq/1
  I_beta/1 -> Mux/4

== system PMSM_RobotKinematics/PMSM5/Park_inv ==
  iq : Inport
  id : Inport  Port=2
  Theta : Inport  Port=3
  Fcn : Fcn  Expr=sin(u)
  Fcn1 : Fcn  Expr=cos(u)
  Gain : Gain  SaturateOnIntegerOverflow=on  OutDataTypeStr=Inherit: Same as input  ParamDataTypeStr=Inherit: Same as input
  Gain1 : Gain  SaturateOnIntegerOverflow=on  OutDataTypeStr=Inherit: Same as input  ParamDataTypeStr=Inherit: Same as input
  Mux : Mux  Inputs=[1 1 1 1]
  i_alpha : Fcn  Expr=u[1]*u[4]-u[2]*u[3]
  i_beta : Fcn  Expr=u[2]*u[4]+u[1]*u[3]
  I_apha : Outport  InitialOutput=0
  I_beta : Outport  Port=2  InitialOutput=0
  wires:
  Fcn/1 -> Mux/2
  Fcn1/1 -> Mux/1
  Theta/1 -> Fcn1/1, Fcn/1
  Mux/1 -> i_beta/1, i_alpha/1
  iq/1 -> Mux/3
  i_beta/1 -> Gain1/1
  i_alpha/1 -> Gain/1
  Gain/1 -> I_apha/1
  Gain1/1 -> I_beta/1
  id/1 -> Mux/4

== system PMSM_RobotKinematics/PMSM5/iqref ==
  In_1 : Inport
  Integral : TransferFcn  Numerator=[I]  Denominator=[1 0]
  Proportional : Gain  Gain=P  SaturateOnIntegerOverflow=on  OutDataTypeStr=Inherit: Same as input  ParamDataTypeStr=Inherit: Same as input
  Saturation : Saturate  UpperLimit=max  LowerLimit=min
  Sum : Sum  SaturateOnIntegerOverflow=on  InputSameDT=on  OutDataTypeStr=Inherit: Same as first input
  Out_1 : Outport  InitialOutput=0
  wires:
  Integral/1 -> Sum/2
  In_1/1 -> Integral/1, Proportional/1
  Proportional/1 -> Sum/1
  Sum/1 -> Saturation/1
  Saturation/1 -> Out_1/1

== system PMSM_RobotKinematics/PMSM5/iqref1 ==
  In_1 : Inport
  Integral : TransferFcn  Numerator=[I]  Denominator=[1 0]
  Proportional : Gain  Gain=P  SaturateOnIntegerOverflow=on  OutDataTypeStr=Inherit: Same as input  ParamDataTypeStr=Inherit: Same as input
  Saturation : Saturate  UpperLimit=max  LowerLimit=min
  Sum : Sum  SaturateOnIntegerOverflow=on  InputSameDT=on  OutDataTypeStr=Inherit: Same as first input
  Out_1 : Outport  InitialOutput=0
  wires:
  Saturation/1 -> Out_1/1
  Sum/1 -> Saturation/1
  Proportional/1 -> Sum/1
  In_1/1 -> Proportional/1, Integral/1
  Integral/1 -> Sum/2

== system PMSM_RobotKinematics/PMSM5/iqref2 ==
  In_1 : Inport
  Integral : TransferFcn  Numerator=[I]  Denominator=[1 0]
  Proportional : Gain  Gain=P  SaturateOnIntegerOverflow=on  OutDataTypeStr=Inherit: Same as input  ParamDataTypeStr=Inherit: Same as input
  Saturation : Saturate  UpperLimit=max  LowerLimit=min
  Sum : Sum  SaturateOnIntegerOverflow=on  InputSameDT=on  OutDataTypeStr=Inherit: Same as first input
  Out_1 : Outport  InitialOutput=0
  wires:
  Saturation/1 -> Out_1/1
  Sum/1 -> Saturation/1
  Proportional/1 -> Sum/1
  In_1/1 -> Proportional/1, Integral/1
  Integral/1 -> Sum/2

== system PMSM_RobotKinematics/PMSM5/iqref3 ==
  In_1 : Inport
  Integral : TransferFcn  Numerator=[I]  Denominator=[1 0]
  Proportional : Gain  Gain=P  SaturateOnIntegerOverflow=on  OutDataTypeStr=Inherit: Same as input  ParamDataTypeStr=Inherit: Same as input
  Saturation : Saturate  UpperLimit=max  LowerLimit=min
  Sum : Sum  SaturateOnIntegerOverflow=on  InputSameDT=on  OutDataTypeStr=Inherit: Same as first input
  Out_1 : Outport  InitialOutput=0
  wires:
  Integral/1 -> Sum/2
  In_1/1 -> Integral/1, Proportional/1
  Proportional/1 -> Sum/1
  Sum/1 -> Saturation/1
  Saturation/1 -> Out_1/1

== system PMSM_RobotKinematics/PMSM6/Clarke ==
  is_abc : Inport
  Gain : Gain  Gain=sqrt(3/2)  SaturateOnIntegerOverflow=on  OutDataTypeStr=Inherit: Same as input  ParamDataTypeStr=Inherit: Same as input
  Gain1 : Gain  Gain=sqrt(2)/2  SaturateOnIntegerOverflow=on  OutDataTypeStr=Inherit: Same as input  ParamDataTypeStr=Inherit: Same as input
  Mux : Mux  Inputs=[3]
  i_alpha : Fcn  Expr=u[1]
  i_beta : Fcn  Expr=u[1]+2*u[2]
  I_alpha : Outport  InitialOutput=0
  I_beta : Outport  Port=2  InitialOutput=0
  wires:
  Gain1/1 -> I_beta/1
  Gain/1 -> I_alpha/1
  i_alpha/1 -> Gain/1
  i_beta/1 -> Gain1/1
  is_abc/1 -> Mux/1
  Mux/1 -> i_alpha/1, i_beta/1

== system PMSM_RobotKinematics/PMSM6/Clarke_inv ==
  Valpha : Inport
  Vbeta : Inport  Port=2
  Fcn : Fcn  Expr=-u[1]/2+1.73205081*u[2]/2
  Fcn1 : Fcn  Expr=-u[1]/2-1.73205081*u[2]/2
  Gain1 : Gain  Gain=sqrt(2/3)  SaturateOnIntegerOverflow=on  OutDataTypeStr=Inherit: Same as input  ParamDataTypeStr=Inherit: Same as input
  Gain2 : Gain  Gain=sqrt(2/3)  SaturateOnIntegerOverflow=on  OutDataTypeStr=Inherit: Same as input  ParamDataTypeStr=Inherit: Same as input
  Gain3 : Gain  Gain=sqrt(2/3)  SaturateOnIntegerOverflow=on  OutDataTypeStr=Inherit: Same as input  ParamDataTypeStr=Inherit: Same as input
  Mux : Mux  Inputs=2
  Va : Outport
  Vb : Outport  Port=2
  Vc : Outport  Port=3
  wires:
  Gain3/1 -> Vc/1
  Gain2/1 -> Vb/1
  Gain1/1 -> Va/1
  Vbeta/1 -> Mux/2
  Valpha/1 -> Gain1/1, Mux/1
  Fcn1/1 -> Gain3/1
  Fcn/1 -> Gain2/1
  Mux/1 -> Fcn1/1, Fcn/1

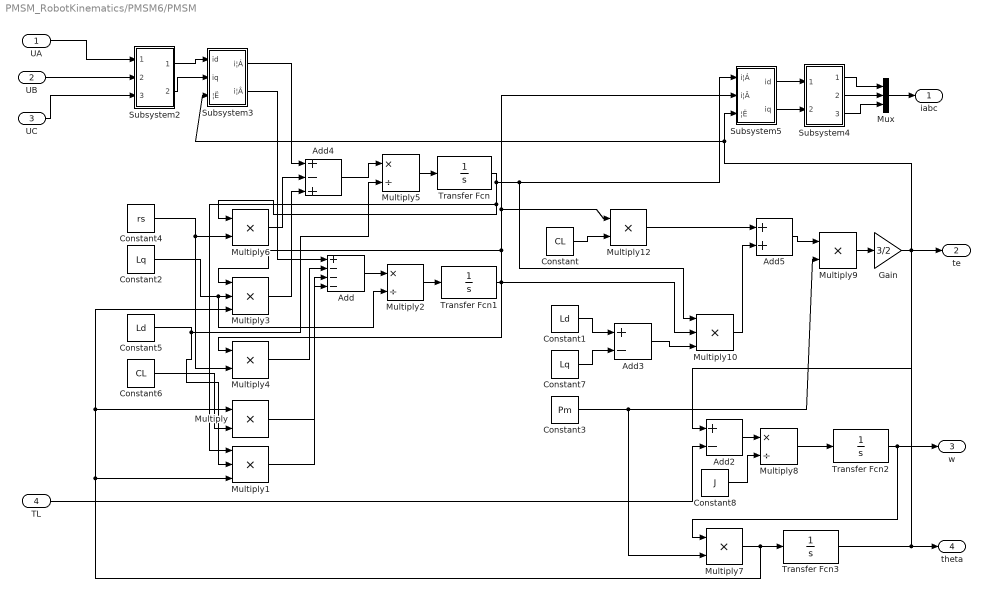
== system PMSM_RobotKinematics/PMSM6/PMSM ==
  UA : Inport
  UB : Inport  Port=2
  UC : Inport  Port=3
  TL : Inport  Port=4
  Add : Sum  Inputs=+---  SaturateOnIntegerOverflow=on  OutDataTypeStr=Inherit: Same as first input
  Add2 : Sum  Inputs=+-  SaturateOnIntegerOverflow=on  InputSameDT=on  OutDataTypeStr=Inherit: Same as first input
  Add3 : Sum  Inputs=+-  SaturateOnIntegerOverflow=on  InputSameDT=on  OutDataTypeStr=Inherit: Same as first input
  Add4 : Sum  Inputs=+-+  SaturateOnIntegerOverflow=on  InputSameDT=on  OutDataTypeStr=Inherit: Same as first input
  Add5 : Sum  SaturateOnIntegerOverflow=on  InputSameDT=on  OutDataTypeStr=Inherit: Same as first input
  Constant : Constant  Value=CL
  Constant1 : Constant  Value=Ld
  Constant2 : Constant  Value=Lq
  Constant3 : Constant  Value=Pm
  Constant4 : Constant  Value=rs
  Constant5 : Constant  Value=Ld
  Constant6 : Constant  Value=CL
  Constant7 : Constant  Value=Lq
  Constant8 : Constant  Value=J
  Gain : Gain  Gain=3/2  SaturateOnIntegerOverflow=on  OutDataTypeStr=Inherit: Same as input  ParamDataTypeStr=Inherit: Same as input
  Multiply{,4,6..7,9,12} (6 alike) : Product  Inputs=**  SaturateOnIntegerOverflow=on  OutDataTypeStr=Inherit: Same as first input
  Multiply1 : Product  Inputs=***  SaturateOnIntegerOverflow=on  OutDataTypeStr=Inherit: Same as first input
  Multiply10 : Product  Inputs=***  SaturateOnIntegerOverflow=on  OutDataTypeStr=Inherit: Same as first input
  Multiply2 : Product  Inputs=*/  SaturateOnIntegerOverflow=on  OutDataTypeStr=Inherit: Same as first input
  Multiply3 : Product  Inputs=***  SaturateOnIntegerOverflow=on  OutDataTypeStr=Inherit: Same as first input
  Multiply5 : Product  Inputs=*/  SaturateOnIntegerOverflow=on  OutDataTypeStr=Inherit: Same as first input
  Multiply8 : Product  Inputs=*/  SaturateOnIntegerOverflow=on  OutDataTypeStr=Inherit: Same as first input
  Mux : Mux  Inputs=3
  Subsystem2 : Subsystem  mask(hao){}
      mask help: 3/2
      mask Help: no
      mask Display: disp('3/2')
  Subsystem3 : Subsystem  mask(2/2){}
      mask help: qdtoMT
      mask Help: none
  Subsystem4 : Subsystem  mask(hao){}
      mask help: 2/3
      mask Help: npi
      mask Display: disp('2/3')
  Subsystem5 : Subsystem  mask(2/2){}
      mask help: mt-todq
      mask Help: no
  Transfer Fcn : TransferFcn  Denominator=[1 0]  AbsoluteTolerance=1e-3
  Transfer Fcn1 : TransferFcn  Denominator=[1 0]
  Transfer Fcn2 : TransferFcn  Denominator=[1 0]
  Transfer Fcn3 : TransferFcn  Denominator=[1 0]
  iabc : Outport
  te : Outport  Port=2
  w : Outport  Port=3
  theta : Outport  Port=4
  wires:
  UB/1 -> Subsystem2/2(In2)
  UA/1 -> Subsystem2/1(In1)
  Subsystem4/2(Out2) -> Mux/2
  Subsystem4/1(Out1) -> Mux/1
  Gain/1 -> Add2/1, te/1
  Transfer Fcn3/1 -> theta/1, Subsystem3/3(¦Ë), Subsystem5/3(¦Ë)
  UC/1 -> Subsystem2/3(In3)
  Multiply8/1 -> Transfer Fcn2/1
  Mux/1 -> iabc/1
  Subsystem4/3(Out3) -> Mux/3
  Multiply9/1 -> Gain/1
  Add5/1 -> Multiply9/1
  Transfer Fcn2/1 -> w/1, Multiply7/1
  Add3/1 -> Multiply10/3
  Constant/1 -> Multiply12/2
  Multiply7/1 -> Multiply1/3, Multiply/1, Multiply3/3, Transfer Fcn3/1
  Constant6/1 -> Multiply/2
  Constant5/1 -> Multiply5/2, Multiply1/2
  Constant2/1 -> Multiply2/2, Multiply3/2
  Transfer Fcn1/1 -> Multiply10/2, Multiply4/1, Subsystem5/2(i¦Â), Multiply12/1, Multiply3/1
  Constant4/1 -> Multiply4/2, Multiply6/2
  Transfer Fcn/1 -> Subsystem5/1(i¦Á), Multiply10/1, Multiply1/1, Multiply6/1
  Subsystem2/1(Out1) -> Subsystem3/1(id)
  Subsystem2/2(Out2) -> Subsystem3/2(iq)
  Subsystem3/1(i¦Á) -> Add4/1
  Multiply6/1 -> Add4/2
  Multiply3/1 -> Add4/3
  Add4/1 -> Multiply5/1
  Subsystem3/2(i¦Â) -> Add/1
  Add/1 -> Multiply2/1
  Multiply4/1 -> Add/2
  Multiply/1 -> Add/3
  Multiply1/1 -> Add/4
  Constant1/1 -> Add3/1
  Constant7/1 -> Add3/2
  Multiply12/1 -> Add5/1
  Multiply10/1 -> Add5/2
  Constant3/1 -> Multiply9/2, Multiply7/2
  Subsystem5/1(id) -> Subsystem4/1(In1)
  Subsystem5/2(iq) -> Subsystem4/2(In3)
  Add2/1 -> Multiply8/1
  Constant8/1 -> Multiply8/2
  TL/1 -> Add2/2
  Multiply5/1 -> Transfer Fcn/1
  Multiply2/1 -> Transfer Fcn1/1

== system PMSM_RobotKinematics/PMSM6/Park ==
  I_alpha : Inport
  I_beta : Inport  Port=2
  Theta : Inport  Port=3
  Fcn : Fcn  Expr=sin(u)
  Fcn1 : Fcn  Expr=cos(u)
  Gain : Gain  SaturateOnIntegerOverflow=on  OutDataTypeStr=Inherit: Same as input  ParamDataTypeStr=Inherit: Same as input
  Gain1 : Gain  SaturateOnIntegerOverflow=on  OutDataTypeStr=Inherit: Same as input  ParamDataTypeStr=Inherit: Same as input
  Mux : Mux  Inputs=[1 1 1 1]
  id : Fcn  Expr=u[1]*u[3]+u[2]*u[4]
  iq : Fcn  Expr=-u[2]*u[3]+u[1]*u[4]
  Id : Outport  InitialOutput=0
  Iq : Outport  Port=2  InitialOutput=0
  wires:
  I_beta/1 -> Mux/4
  Gain1/1 -> Iq/1
  Gain/1 -> Id/1
  id/1 -> Gain/1
  iq/1 -> Gain1/1
  I_alpha/1 -> Mux/3
  Mux/1 -> id/1, iq/1
  Theta/1 -> Fcn/1, Fcn1/1
  Fcn1/1 -> Mux/1
  Fcn/1 -> Mux/2

== system PMSM_RobotKinematics/PMSM6/Park_inv ==
  iq : Inport
  id : Inport  Port=2
  Theta : Inport  Port=3
  Fcn : Fcn  Expr=sin(u)
  Fcn1 : Fcn  Expr=cos(u)
  Gain : Gain  SaturateOnIntegerOverflow=on  OutDataTypeStr=Inherit: Same as input  ParamDataTypeStr=Inherit: Same as input
  Gain1 : Gain  SaturateOnIntegerOverflow=on  OutDataTypeStr=Inherit: Same as input  ParamDataTypeStr=Inherit: Same as input
  Mux : Mux  Inputs=[1 1 1 1]
  i_alpha : Fcn  Expr=u[1]*u[4]-u[2]*u[3]
  i_beta : Fcn  Expr=u[2]*u[4]+u[1]*u[3]
  I_apha : Outport  InitialOutput=0
  I_beta : Outport  Port=2  InitialOutput=0
  wires:
  id/1 -> Mux/4
  Gain1/1 -> I_beta/1
  Gain/1 -> I_apha/1
  i_alpha/1 -> Gain/1
  i_beta/1 -> Gain1/1
  iq/1 -> Mux/3
  Mux/1 -> i_alpha/1, i_beta/1
  Theta/1 -> Fcn/1, Fcn1/1
  Fcn1/1 -> Mux/1
  Fcn/1 -> Mux/2

== system PMSM_RobotKinematics/PMSM6/iqref ==
  In_1 : Inport
  Integral : TransferFcn  Numerator=[I]  Denominator=[1 0]
  Proportional : Gain  Gain=P  SaturateOnIntegerOverflow=on  OutDataTypeStr=Inherit: Same as input  ParamDataTypeStr=Inherit: Same as input
  Saturation : Saturate  UpperLimit=max  LowerLimit=min
  Sum : Sum  SaturateOnIntegerOverflow=on  InputSameDT=on  OutDataTypeStr=Inherit: Same as first input
  Out_1 : Outport  InitialOutput=0
  wires:
  Saturation/1 -> Out_1/1
  Sum/1 -> Saturation/1
  Proportional/1 -> Sum/1
  In_1/1 -> Proportional/1, Integral/1
  Integral/1 -> Sum/2

== system PMSM_RobotKinematics/PMSM6/iqref1 ==
  In_1 : Inport
  Integral : TransferFcn  Numerator=[I]  Denominator=[1 0]
  Proportional : Gain  Gain=P  SaturateOnIntegerOverflow=on  OutDataTypeStr=Inherit: Same as input  ParamDataTypeStr=Inherit: Same as input
  Saturation : Saturate  UpperLimit=max  LowerLimit=min
  Sum : Sum  SaturateOnIntegerOverflow=on  InputSameDT=on  OutDataTypeStr=Inherit: Same as first input
  Out_1 : Outport  InitialOutput=0
  wires:
  Integral/1 -> Sum/2
  In_1/1 -> Integral/1, Proportional/1
  Proportional/1 -> Sum/1
  Sum/1 -> Saturation/1
  Saturation/1 -> Out_1/1

== system PMSM_RobotKinematics/PMSM6/iqref2 ==
  In_1 : Inport
  Integral : TransferFcn  Numerator=[I]  Denominator=[1 0]
  Proportional : Gain  Gain=P  SaturateOnIntegerOverflow=on  OutDataTypeStr=Inherit: Same as input  ParamDataTypeStr=Inherit: Same as input
  Saturation : Saturate  UpperLimit=max  LowerLimit=min
  Sum : Sum  SaturateOnIntegerOverflow=on  InputSameDT=on  OutDataTypeStr=Inherit: Same as first input
  Out_1 : Outport  InitialOutput=0
  wires:
  Integral/1 -> Sum/2
  In_1/1 -> Integral/1, Proportional/1
  Proportional/1 -> Sum/1
  Sum/1 -> Saturation/1
  Saturation/1 -> Out_1/1

== system PMSM_RobotKinematics/PMSM6/iqref3 ==
  In_1 : Inport
  Integral : TransferFcn  Numerator=[I]  Denominator=[1 0]
  Proportional : Gain  Gain=P  SaturateOnIntegerOverflow=on  OutDataTypeStr=Inherit: Same as input  ParamDataTypeStr=Inherit: Same as input
  Saturation : Saturate  UpperLimit=max  LowerLimit=min
  Sum : Sum  SaturateOnIntegerOverflow=on  InputSameDT=on  OutDataTypeStr=Inherit: Same as first input
  Out_1 : Outport  InitialOutput=0
  wires:
  Saturation/1 -> Out_1/1
  Sum/1 -> Saturation/1
  Proportional/1 -> Sum/1
  In_1/1 -> Proportional/1, Integral/1
  Integral/1 -> Sum/2

== system PMSM_RobotKinematics/Robot/Joint1 ==
  note: 初始角度
  note: 初始角度
  BaseBracket_1_RIGID : Subsystem
  PS Add : fl_lib/Physical Signals/Functions/PS Add
  PS Constant : fl_lib/Physical Signals/Sources/PS Constant  constant=-pi/2
  PS Constant1 : fl_lib/Physical Signals/Sources/PS Constant  constant=-pi/2
  PS Subtract1 : fl_lib/Physical Signals/Functions/PS Subtract
      settings: SourceProductName=Simscape
  Revolute1 : sm_lib/Joints/Revolute Joint  SenseConstraintForce=off  SenseConstraintForceX=off  SenseConstraintForceY=off  SenseConstraintForceZ=off  SenseConstraintTorque=off  SenseConstraintTorqueX=off  SenseConstraintTorqueY=off  SenseConstraintTorqueZ=off  SenseTotalForce=off  SenseTotalForceX=off  SenseTotalForceY=off  SenseTotalForceZ=off  SenseTotalTorque=off  SenseTotalTorqueX=off  SenseTotalTorqueY=off  SenseTotalTorqueZ=off  CompositeWrenchDir=FollowerOnBase  CompositeWrenchFrame=BaseFrame  EquilibriumPosition=0  EquilibriumPositionUnits=rad  SpringStiffness=0  SpringStiffnessUnits=N*m/rad  DampingCoefficient=0  DampingCoefficientUnits=N*m/(rad/s)  TorqueActuationMode=ComputedTorque  MotionActuationMode=InputMotion  SensePosition=on  SenseVelocity=on  SenseAcceleration=off  SenseTorqueForce=off  PositionTargetSpecify=on  PositionTargetPriority=Low  PositionTargetValue=smiData.RevoluteJoint(2).Rz.Pos  PositionTargetValueUnits=deg  VelocityTargetSpecify=off  VelocityTargetPriority=High  VelocityTargetValue=0  VelocityTargetValueUnits=deg/s
  BaseConn : PMIOPort  Side=Left
  Motion1 : PMIOPort  Port=2  Side=Left
  q1 : PMIOPort  Port=3  Side=Right
  w1 : PMIOPort  Port=4  Side=Right
  Conn1 : PMIOPort  Port=5  Side=Right
  connections:
  BaseBracket_1_RIGID/RConn1 -- Revolute1/LConn1
  PS Add/RConn1 -- Revolute1/LConn2
  Conn1/RConn1 -- Revolute1/RConn1
  BaseBracket_1_RIGID/LConn1 -- BaseConn/RConn1
  PS Subtract1/LConn1 -- Revolute1/RConn2
  w1/RConn1 -- Revolute1/RConn3
  PS Add/LConn2 -- Motion1/RConn1
  PS Add/LConn1 -- PS Constant/RConn1
  PS Constant1/RConn1 -- PS Subtract1/LConn2
  PS Subtract1/RConn1 -- q1/RConn1

== system PMSM_RobotKinematics/Robot/Joint2 ==
  note: 初始角度
  note: 初始角度
  Link1_2_RIGID : Subsystem
  PS Add : fl_lib/Physical Signals/Functions/PS Add
  PS Constant1 : fl_lib/Physical Signals/Sources/PS Constant  constant=-pi/2
  PS Constant2 : fl_lib/Physical Signals/Sources/PS Constant  constant=-pi/2
  PS Subtract1 : fl_lib/Physical Signals/Functions/PS Subtract
      settings: SourceProductName=Simscape
  Revolute : sm_lib/Joints/Revolute Joint  SenseConstraintForce=off  SenseConstraintForceX=off  SenseConstraintForceY=off  SenseConstraintForceZ=off  SenseConstraintTorque=off  SenseConstraintTorqueX=off  SenseConstraintTorqueY=off  SenseConstraintTorqueZ=off  SenseTotalForce=off  SenseTotalForceX=off  SenseTotalForceY=off  SenseTotalForceZ=off  SenseTotalTorque=off  SenseTotalTorqueX=off  SenseTotalTorqueY=off  SenseTotalTorqueZ=off  CompositeWrenchDir=FollowerOnBase  CompositeWrenchFrame=BaseFrame  EquilibriumPosition=0  EquilibriumPositionUnits=rad  SpringStiffness=0  SpringStiffnessUnits=N*m/rad  DampingCoefficient=0  DampingCoefficientUnits=N*m/(rad/s)  TorqueActuationMode=ComputedTorque  MotionActuationMode=InputMotion  SensePosition=on  SenseVelocity=on  SenseAcceleration=off  SenseTorqueForce=off  PositionTargetSpecify=on  PositionTargetPriority=Low  PositionTargetValue=smiData.RevoluteJoint(1).Rz.Pos  PositionTargetValueUnits=deg  VelocityTargetSpecify=off  VelocityTargetPriority=High  VelocityTargetValue=0  VelocityTargetValueUnits=deg/s
  Conn1 : PMIOPort  Side=Left
  q2 : PMIOPort  Port=2  Side=Right
  Motion2 : PMIOPort  Port=3  Side=Left
  w2 : PMIOPort  Port=4  Side=Right
  Conn2 : PMIOPort  Port=5  Side=Right
  connections:
  PS Add/LConn2 -- Motion2/RConn1
  Link1_2_RIGID/LConn1 -- Conn1/RConn1
  Link1_2_RIGID/RConn1 -- Revolute/LConn1
  Conn2/RConn1 -- Revolute/RConn1
  Revolute/RConn2 -- PS Subtract1/LConn1
  Revolute/RConn3 -- w2/RConn1
  PS Constant1/RConn1 -- PS Add/LConn1
  PS Add/RConn1 -- Revolute/LConn2
  PS Subtract1/RConn1 -- q2/RConn1
  PS Constant2/RConn1 -- PS Subtract1/LConn2

== system PMSM_RobotKinematics/Robot/Joint3 ==
  note: 初始角度
  note: 初始角度
  Link2_2_RIGID : Subsystem
  PS Add : fl_lib/Physical Signals/Functions/PS Add
  PS Constant1 : fl_lib/Physical Signals/Sources/PS Constant  constant=0
  PS Constant2 : fl_lib/Physical Signals/Sources/PS Constant  constant=0
  PS Subtract1 : fl_lib/Physical Signals/Functions/PS Subtract
      settings: SourceProductName=Simscape
  Revolute2 : sm_lib/Joints/Revolute Joint  SenseConstraintForce=off  SenseConstraintForceX=off  SenseConstraintForceY=off  SenseConstraintForceZ=off  SenseConstraintTorque=off  SenseConstraintTorqueX=off  SenseConstraintTorqueY=off  SenseConstraintTorqueZ=off  SenseTotalForce=off  SenseTotalForceX=off  SenseTotalForceY=off  SenseTotalForceZ=off  SenseTotalTorque=off  SenseTotalTorqueX=off  SenseTotalTorqueY=off  SenseTotalTorqueZ=off  CompositeWrenchDir=FollowerOnBase  CompositeWrenchFrame=BaseFrame  EquilibriumPosition=0  EquilibriumPositionUnits=rad  SpringStiffness=0  SpringStiffnessUnits=N*m/rad  DampingCoefficient=0  DampingCoefficientUnits=N*m/(rad/s)  TorqueActuationMode=ComputedTorque  MotionActuationMode=InputMotion  SensePosition=on  SenseVelocity=on  SenseAcceleration=off  SenseTorqueForce=off  PositionTargetSpecify=on  PositionTargetPriority=Low  PositionTargetValue=smiData.RevoluteJoint(3).Rz.Pos  PositionTargetValueUnits=deg  VelocityTargetSpecify=off  VelocityTargetPriority=High  VelocityTargetValue=0  VelocityTargetValueUnits=deg/s
  Conn2 : PMIOPort  Side=Left
  Motion2 : PMIOPort  Port=2  Side=Left
  q3 : PMIOPort  Port=3  Side=Right
  w3 : PMIOPort  Port=4  Side=Right
  Conn3 : PMIOPort  Port=5  Side=Right
  connections:
  Link2_2_RIGID/RConn1 -- Revolute2/LConn1
  Link2_2_RIGID/LConn1 -- Conn2/RConn1
  PS Add/RConn1 -- Revolute2/LConn2
  PS Add/LConn1 -- PS Constant1/RConn1
  Conn3/RConn1 -- Revolute2/RConn1
  PS Constant2/RConn1 -- PS Subtract1/LConn2
  PS Subtract1/RConn1 -- q3/RConn1
  PS Subtract1/LConn1 -- Revolute2/RConn2
  w3/RConn1 -- Revolute2/RConn3
  Motion2/RConn1 -- PS Add/LConn2

== system PMSM_RobotKinematics/Robot/Joint4 ==
  note: 初始角度
  note: 初始角度
  Link3_1_RIGID : Subsystem
  PS Add : fl_lib/Physical Signals/Functions/PS Add
  PS Constant1 : fl_lib/Physical Signals/Sources/PS Constant  constant=0
  PS Constant2 : fl_lib/Physical Signals/Sources/PS Constant  constant=0
  PS Subtract1 : fl_lib/Physical Signals/Functions/PS Subtract
      settings: SourceProductName=Simscape
  Revolute3 : sm_lib/Joints/Revolute Joint  SenseConstraintForce=off  SenseConstraintForceX=off  SenseConstraintForceY=off  SenseConstraintForceZ=off  SenseConstraintTorque=off  SenseConstraintTorqueX=off  SenseConstraintTorqueY=off  SenseConstraintTorqueZ=off  SenseTotalForce=off  SenseTotalForceX=off  SenseTotalForceY=off  SenseTotalForceZ=off  SenseTotalTorque=off  SenseTotalTorqueX=off  SenseTotalTorqueY=off  SenseTotalTorqueZ=off  CompositeWrenchDir=FollowerOnBase  CompositeWrenchFrame=BaseFrame  EquilibriumPosition=0  EquilibriumPositionUnits=rad  SpringStiffness=0  SpringStiffnessUnits=N*m/rad  DampingCoefficient=0  DampingCoefficientUnits=N*m/(rad/s)  TorqueActuationMode=ComputedTorque  MotionActuationMode=InputMotion  SensePosition=on  SenseVelocity=on  SenseAcceleration=off  SenseTorqueForce=off  PositionTargetSpecify=on  PositionTargetPriority=Low  PositionTargetValue=smiData.RevoluteJoint(4).Rz.Pos  PositionTargetValueUnits=deg  VelocityTargetSpecify=off  VelocityTargetPriority=High  VelocityTargetValue=0  VelocityTargetValueUnits=deg/s
  Conn3 : PMIOPort  Side=Left
  Motion4 : PMIOPort  Port=2  Side=Left
  q4 : PMIOPort  Port=3  Side=Right
  w4 : PMIOPort  Port=4  Side=Right
  Conn4 : PMIOPort  Port=5  Side=Right
  connections:
  PS Add/RConn1 -- Revolute3/LConn2
  Link3_1_RIGID/RConn1 -- Revolute3/LConn1
  Link3_1_RIGID/LConn1 -- Conn3/RConn1
  PS Subtract1/LConn1 -- Revolute3/RConn2
  PS Add/LConn2 -- Motion4/RConn1
  PS Subtract1/RConn1 -- q4/RConn1
  PS Constant2/RConn1 -- PS Subtract1/LConn2
  Conn4/RConn1 -- Revolute3/RConn1
  PS Add/LConn1 -- PS Constant1/RConn1
  w4/RConn1 -- Revolute3/RConn3

== system PMSM_RobotKinematics/Robot/Joint5 ==
  note: 初始角度
  note: 初始角度
  Link4_1_RIGID : Subsystem
  PS Add : fl_lib/Physical Signals/Functions/PS Add
  PS Constant1 : fl_lib/Physical Signals/Sources/PS Constant  constant=pi/2
  PS Constant2 : fl_lib/Physical Signals/Sources/PS Constant  constant=pi/2
  PS Subtract1 : fl_lib/Physical Signals/Functions/PS Subtract
      settings: SourceProductName=Simscape
  Revolute5 : sm_lib/Joints/Revolute Joint  SenseConstraintForce=off  SenseConstraintForceX=off  SenseConstraintForceY=off  SenseConstraintForceZ=off  SenseConstraintTorque=off  SenseConstraintTorqueX=off  SenseConstraintTorqueY=off  SenseConstraintTorqueZ=off  SenseTotalForce=off  SenseTotalForceX=off  SenseTotalForceY=off  SenseTotalForceZ=off  SenseTotalTorque=off  SenseTotalTorqueX=off  SenseTotalTorqueY=off  SenseTotalTorqueZ=off  CompositeWrenchDir=FollowerOnBase  CompositeWrenchFrame=BaseFrame  EquilibriumPosition=0  EquilibriumPositionUnits=rad  SpringStiffness=0  SpringStiffnessUnits=N*m/rad  DampingCoefficient=0  DampingCoefficientUnits=N*m/(rad/s)  TorqueActuationMode=ComputedTorque  MotionActuationMode=InputMotion  SensePosition=on  SenseVelocity=on  SenseAcceleration=off  SenseTorqueForce=off  PositionTargetSpecify=on  PositionTargetPriority=Low  PositionTargetValue=smiData.RevoluteJoint(5).Rz.Pos  PositionTargetValueUnits=deg  VelocityTargetSpecify=off  VelocityTargetPriority=High  VelocityTargetValue=0  VelocityTargetValueUnits=deg/s
  Conn4 : PMIOPort  Side=Left
  Motion5 : PMIOPort  Port=2  Side=Left
  q5 : PMIOPort  Port=3  Side=Right
  w5 : PMIOPort  Port=4  Side=Right
  Conn5 : PMIOPort  Port=5  Side=Right
  connections:
  Link4_1_RIGID/RConn1 -- Revolute5/LConn1
  PS Add/RConn1 -- Revolute5/LConn2
  Link4_1_RIGID/LConn1 -- Conn4/RConn1
  PS Subtract1/LConn1 -- Revolute5/RConn2
  PS Add/LConn2 -- Motion5/RConn1
  PS Subtract1/RConn1 -- q5/RConn1
  PS Constant2/RConn1 -- PS Subtract1/LConn2
  Conn5/RConn1 -- Revolute5/RConn1
  PS Constant1/RConn1 -- PS Add/LConn1
  w5/RConn1 -- Revolute5/RConn3
